simulink model "Coupeller"  (R2024b)
settings: Solver=VariableStepAuto  StartTime=0.0  StopTime=1  RelTol=1e-3
libraries: simrfV2util1 x3, simrfV2elements x1, simrfV2sources1 x1

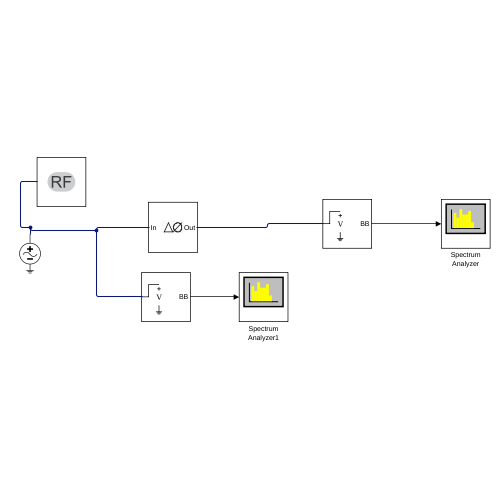
[thumbnail: Simulink's stored preview of the top-level diagram]
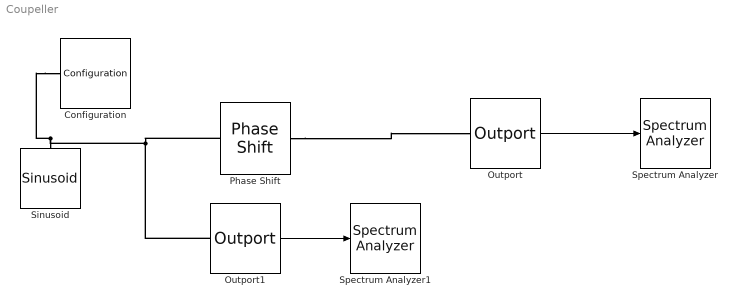
== system Coupeller ==
  Configuration : simrfV2util1/Configuration  AutoFreq=on  Tones=[] Hz  Harmonics=[]  NormalizeCarrierPower=on  SolverType=Auto  UseCCode=on  StepSize=1e-6 s  AddNoise=on  defaultRNG=on  Seed=0  Temperature=290.0 K  SolverDelFlag=0  AbsTol=1e-6  RelTol=1e-3  MaxIter=10  ErrorEstimationType=2-norm over all variables  EnableInterpFilter=on  HiddenFIRfilterControllerParam=off  SmallSignalApprox=off  AllSimFreqs=on  SimFreqs=[] Hz  SimFreqsInternal=[]  SamplesPerFrame=1
  Outport : simrfV2util1/Outport  SensorType=Ideal voltage  OutputFormat=Complex Baseband  CarrierFreq=1 GHz  ZL=Inf  InternalGrounding=on  StepSize=1e-6 s  AutoStep=on  HalfPolyphaseLength=12
  Outport1 : simrfV2util1/Outport  SensorType=Ideal voltage  OutputFormat=Complex Baseband  CarrierFreq=1 GHz  ZL=Inf  InternalGrounding=on  StepSize=1e-6 s  AutoStep=on  HalfPolyphaseLength=12
  Phase Shift : simrfV2elements/Phase Shift  PhaseShift=90 deg  InternalGrounding=on
  Sinusoid : simrfV2sources1/Sinusoid  SineSourceType=Ideal voltage  VO_I=0 V  IO_I=0 A  VO_Q=0 V  IO_Q=0 A  VA_I=5 V  IA_I=0 A  VA_Q=0 V  IA_Q=0 A  Fmod=1 MHz  TD=0 s  CarrierFreq=1 GHz  InternalGrounding=on
  Spectrum Analyzer : SpectrumAnalyzer  Tag=simrfV2util1/Spectrum Analyzer  WindowPosition=[718.000000,121.000000,549.000000,500.000000,]  Visible=on  ScopeFrameLocation=window  Method=Welch  AveragingMethod=Exponential  YLimits=[-151.38927485180284,88.80615695905537]  AllowFFTLengthLessThanSamplesPerUpdate=on
  Spectrum Analyzer1 : SpectrumAnalyzer  Tag=simrfV2util1/Spectrum Analyzer  WindowPosition=[44.000000,116.000000,563.000000,500.000000,]  Visible=on  ScopeFrameLocation=window  Method=Welch  AveragingMethod=Exponential  YLimits=[-269.70130684963397,-70.17570874624015]  AllowFFTLengthLessThanSamplesPerUpdate=on
  wires:
  Outport1/1 -> Spectrum Analyzer1/1
  Outport/1 -> Spectrum Analyzer/1
  connections:
  Configuration/LConn1 -- Outport1/LConn1 -- Phase Shift/LConn1 -- Sinusoid/LConn1
  Phase Shift/RConn1 -- Outport/LConn1
